simulink model "Sim_v18"  (Simulink 8.5)
settings: Solver=ode4  StartTime=0.0  StopTime=300  FixedStep=Ts  RelTol=1e-3
PreLoadFcn:
  | Ts=0.1;
PostLoadFcn:
  | Ts=0.1;
InitFcn:
  | Ts=0.1;
StartFcn:
  | Ts=0.1;
values from neighbouring files (symbols this model uses):
  ctrl_idx = strToIdx(actStr,loadNames)    [Driver_13NFbalanced.m]    (also in Driver_13NFunbalanced.m; Driver_4NFunbalanced.m; Driver_AL0001.m; Driver_Adam.m)
  dbc_idx = strToIdx(dbcStr,loadNames)    [Driver_13NFbalanced.m]    (also in Driver_13NFunbalanced.m; Driver_4NFunbalanced.m; Driver_AL0001.m; Driver_Adam.m)
  Ki_vang = zeros(r,1)    [Driver_4NFunbalanced.m]    (also in ZNset.m = 0.5*Ku/Tu; ZNtune.m = 0; afunc.m; computeK_ZN.m = zeros(1,r))
  Ki_vmag = [f2*ones(3,1); f3*ones(3,1)]    [Driver_4NFunbalanced.m]    (also in ZNset.m = 0.5*Ku/Tu; ZNtune.m = 0; afunc.m = zeros(r,1); computeK_ZN.m = zeros(1,r))
  Kp_vang = zeros(r,1)    [Driver_4NFunbalanced.m]    (also in ZNset.m = 0.4*Ku; ZNtune.m = 0.17; afunc.m; computeK_ZN.m = zeros(1,r))
  Kp_vmag = zeros(r,1)    [Driver_4NFunbalanced.m]    (also in ZNset.m = 0.4*Ku; ZNtune.m = 9.5; afunc.m; computeK_ZN.m = zeros(1,r))
  meas_idx = strToIdx(measStr,busNames)    [Driver_13NFbalanced.m]    (also in Driver_13NFunbalanced.m; Driver_4NFunbalanced.m; Driver_AL0001.m; Driver_Adam.m)
  Sbase = 500    [computePU.m]
  Sinv = 600    [Constraints_update.m]    (also in Driver_13NFbalanced.m = repmat(Sinv_str,1,length(ctrl_idx)/2); Driver_13NFunbalanced.m = repmat(Sinv_str,1,length(ctrl_idx)/2); Driver_4NFunbalanced.m = repmat(Sinv_str,1,length(ctrl_idx)/2); Driver_AL0001.m = repmat(Sinv_str,1,length(ctrl_idx)/2))
  V1base = V1_ph    [computePU.m]
  vang_init_actual = vang_new(4,:)    [Driver_13NFbalanced.m]    (also in Driver_13NFunbalanced.m = vang_new(40,:); Driver_4NFunbalanced.m = vang_new(40,:); Driver_AL0001.m = vang_new(40,:); Driver_Adam.m)
  Vmag_ctrlStart = 60    [Driver_4NFunbalanced.m]    (also in afunc.m = 5; computeK_ZN.m = 5; computeK_ZNplus.m = 5; computeK_way3.m = 5)
  vmag_init_actual = vmag_new(4,:)    [Driver_13NFbalanced.m]    (also in Driver_13NFunbalanced.m = vmag_new(40,:); Driver_4NFunbalanced.m = vmag_new(40,:); Driver_AL0001.m = vmag_new(40,:); Driver_Adam.m)
libraries: opal_lib x2, rtlab x2, rtlab_phasor x1
settings Model: Creator=Jaimie.Swartz  LastModifiedBy=Jaimie.Swartz
settings SolverCC: AlgebraicLoopSolver=LineSearch
settings DataIOCC: SignalLogging=off  DSMLogging=off  VisualizeSimOutput=off
settings DebuggingCC: SolverPrmCheckMsg=warning  FcnCallInpInsideContextMsg=EnableAllAsWarning
settings ConfigurationSet: Description=SimMechanics 2G

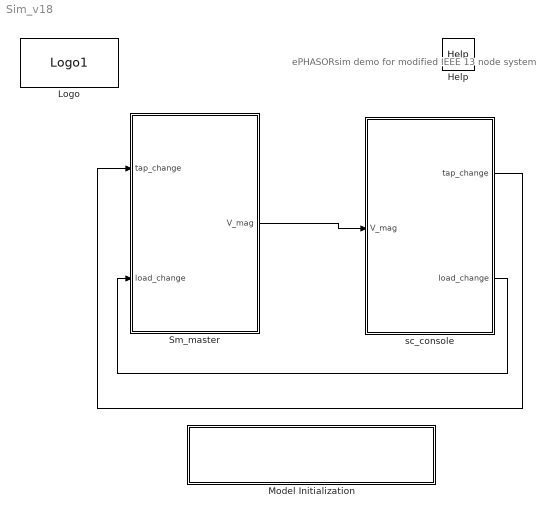
== system Sim_v18 ==
  note: ePHASORsim demo for
      | modified IEEE 13 node system
  Help : opal_lib/Help  docfile=../help/ePH_IEEE13.html
  Logo : opal_lib/Logo1  vide=[]
  Model Initialization : Subsystem  mask(Model Functions){InitFcnX=Ts=0.1;, prel=on, posl=on, inif=on, strf=on}
      mask prompts: InitFcnX "Initialisation"; prel "Preload Function"; posl "PostLoad Function"; inif "InitFcn"; strf "StartFcn"
      mask init:
      | currentBlock = gcb;
      | root = bdroot(currentBlock);
      | 
      | if ~strcmp(get_param(root,'BlockDiagramType'),'library')
      |     if prel==1
      |         set_param(root, 'PreLoadFcn', InitFcnX);
      |     else
      |         set_param(root, 'PreLoadFcn', '');
      |     end
      |     if inif==1
      |         set_param(root, 'InitFcn', InitFcnX);
      |     else
      |         set_param(root, 'InitFcn', '');
      |     end
      |     if strf==1
      |         set_param(root, 'StartFcn', InitFcnX);
      |     else
      |         set_param(root, 'StartFcn', '');
      |     end
      |     if posl==1
      |         set_param(root, 'PostLoadFcn', InitFcnX);
      |     else
      |         set_param(root, 'PostLoadFcn', '');
      |     end
      | end
      | 
      | pos = get_param(currentBlock, 'Position');
      | width = pos(3) - pos(1); height = pos(4) - pos(2);
      | txt = [ upper(root) '\n' '- InitFcn. . . . . '  get_param(root, 'InitFcn') ];
      settings: CopyFcn=set_param(gcb,'LinkStatus','none')
      mask Display: text(5, height*0.5, txt, 'horizontalAlignment', 'left', 'verticalAlignment', 'middle') ;
  Sm_master : Subsystem
  sc_console : Subsystem
  wires:
  Sm_master/1(V_mag) -> sc_console/1(V_mag)
  sc_console/1(tap_change) -> Sm_master/1(tap_change)
  sc_console/2(load_change) -> Sm_master/2(load_change)

== system Sim_v18/Model Initialization ==

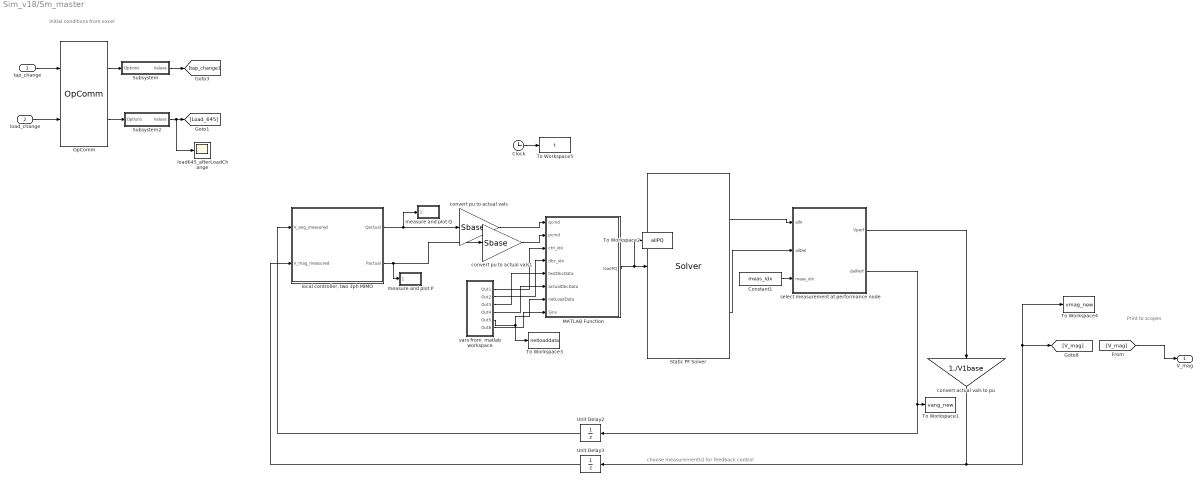
== system Sim_v18/Sm_master ==
  note: Initial conditions from excel
  note: choose measurement(s) for feedback control
  note: Print to scopes
  tap_change : Inport
  load_change : Inport  Port=2
  Clock : Clock
  Constant1 : Constant  Value=meas_idx
  MATLAB Function : MATLAB Function  TreatAsAtomicUnit=on
  OpComm : rtlab/OpComm  nbport=2  groupe_acq=1  subsys_rate=0  st=0  Synchronization=on  Interpolation=on  Threshold=1.0  Missed_Data=off  Sim_Time=off  Samples=off  dynSigOut=off  from_console=1  warning_done=off  writeOpCommFile=off  Offset=off
  Static PF Solver : rtlab_phasor/Solver  epname=System  extension=Excel  xls='impedMod_IEEE13.xls'  raw='4992b.raw'  dyr='4992b.dyr'  cyme='ieee13.sxst'  powerfactory='network.dgs'  builtin=on  cyme_pf=''  cyme_unbalanced=on  lazy_netlist=on  capidir='CAPI'  fmudir='FMU'  capiprefix=capicomp_  fmuprefix=fmucomp_  logging=off  sim_mode=Power-flow and dynamic simulation  pf_max_it=100  pf_tol_v=0.00000001  pf_flat_start=off  pf_smart_start=off  pf_export=on  np=1  exporty=off  dt=Ts  optim_threads=off  perflog_on=off  script_activate_postinit=off  script_postinit_name=''
  Subsystem : Subsystem
  Subsystem2 : Subsystem
  To Workspace1 : ToWorkspace  VariableName=vang_new  SampleTime=-1
      settings: Save2DSignal=2-D array (concatenate along first dimension)
  To Workspace2 : ToWorkspace  VariableName=allPQ  SampleTime=-1
      settings: Save2DSignal=2-D array (concatenate along first dimension)
  To Workspace3 : ToWorkspace  VariableName=netloaddata  SampleTime=-1
      settings: Save2DSignal=2-D array (concatenate along first dimension)
  To Workspace4 : ToWorkspace  VariableName=vmag_new  SampleTime=-1
      settings: Save2DSignal=2-D array (concatenate along first dimension)
  To Workspace5 : ToWorkspace  VariableName=t  SampleTime=-1
      settings: Save2DSignal=2-D array (concatenate along first dimension)
  Unit Delay2 : UnitDelay  InitialCondition=vang_init_actual  SampleTime=Ts
  Unit Delay3 : UnitDelay  InitialCondition=vmag_init_actual  SampleTime=Ts
  convert actual vals to pu : Gain  Gain=1./V1base
  convert pu to actual vals : Gain  Gain=Sbase
  convert pu to actual vals1 : Gain  Gain=Sbase
  load645_afterLoadChange : Scope
      settings: ShowLegends=on  YMin=0.94469  YMax=1.0518  SaveName=ScopeData17
  "local controller, two 3ph MIMO" : Subsystem
  measure and plot P : Subsystem
  measure and plot Q : Subsystem
  select measurement at performance node : MATLAB Function  TreatAsAtomicUnit=on
  vars from  matlab workspace : Subsystem
  V_mag : Outport
  wires:
  tap_change/1 -> OpComm/1
  load_change/1 -> OpComm/2
  [V_mag] -> V_mag/1
  OpComm/1 -> Subsystem/1(Options)
  OpComm/2 -> Subsystem2/1(Options)
  Subsystem/1(Values) -> [tap_change]
  Subsystem2/1(Values) -> load645_afterLoadChange/1, [Load_645]
  convert actual vals to pu/1 -> Unit Delay3/1, To Workspace4/1, [V_mag]
  Unit Delay2/1 -> "local controller, two 3ph MIMO"/1(V_ang_measured)
  Unit Delay3/1 -> "local controller, two 3ph MIMO"/2(V_mag_measured)
  Static PF Solver/1 -> select measurement at performance node/1(allV)
  Static PF Solver/2 -> select measurement at performance node/2(allDel)
  "local controller, two 3ph MIMO"/1(Qactual) -> convert pu to actual vals/1, measure and plot Q/1(Qactual)
  "local controller, two 3ph MIMO"/2(Pactual) -> measure and plot P/1(Pactual), convert pu to actual vals1/1
  MATLAB Function/1(loadPQ) -> To Workspace2/1, Static PF Solver/1
  select measurement at performance node/1(Vperf) -> convert actual vals to pu/1
  select measurement at performance node/2(delPerf) -> Unit Delay2/1, To Workspace1/1
  vars from  matlab workspace/1(Out1) -> MATLAB Function/3(ctrl_idx)
  vars from  matlab workspace/2(Out2) -> MATLAB Function/4(dbc_idx)
  Constant1/1 -> select measurement at performance node/3(meas_idx)
  vars from  matlab workspace/5(Out5) -> To Workspace3/1, MATLAB Function/7(netLoadData)
  convert pu to actual vals/1 -> MATLAB Function/1(qcmd)
  convert pu to actual vals1/1 -> MATLAB Function/2(pcmd)
  Clock/1 -> To Workspace5/1
  vars from  matlab workspace/3(Out3) -> MATLAB Function/5(testDbcData)
  vars from  matlab workspace/4(Out4) -> MATLAB Function/6(actualDbcData)
  vars from  matlab workspace/6(Out6) -> MATLAB Function/8(Sinv)

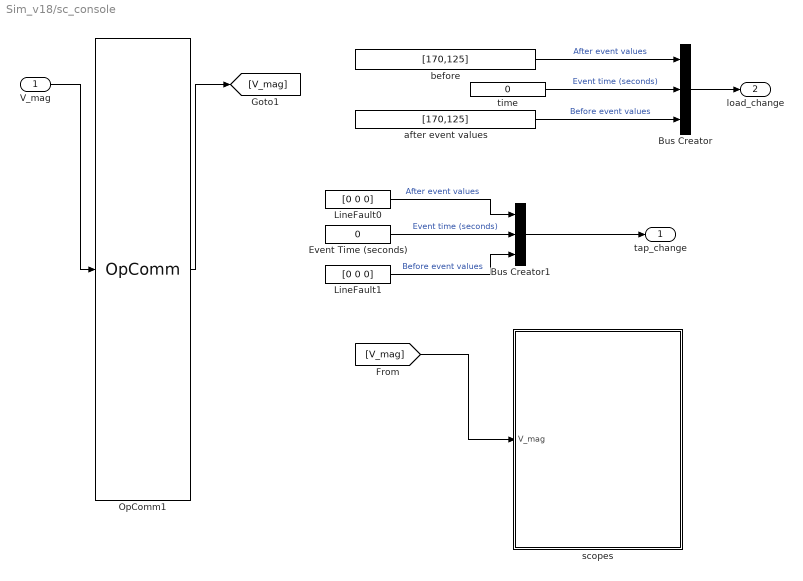
== system Sim_v18/sc_console ==
  V_mag : Inport
  Bus Creator : BusCreator  Inputs=3
  Bus Creator1 : BusCreator  Inputs=3
  Event Time (seconds) : Constant  Value=0
  LineFault0 : Constant  Value=[0 0 0]
  LineFault1 : Constant  Value=[0 0 0]
  OpComm1 : rtlab/OpComm  nbport=1  groupe_acq=1  subsys_rate=0  st=0  Synchronization=on  Interpolation=on  Threshold=1.0  Missed_Data=off  Sim_Time=off  Samples=off  dynSigOut=off  from_console=0  warning_done=off  writeOpCommFile=off  Offset=off
  after event values : Constant  Value=[170,125]
  before : Constant  Value=[170,125]
  scopes : Subsystem
  time : Constant  Value=0
  tap_change : Outport
  load_change : Outport  Port=2
  wires:
  V_mag/1 -> OpComm1/1
  OpComm1/1 -> [V_mag]
  time/1 -> Bus Creator/2  "Event time (seconds)"
  Bus Creator/1 -> load_change/1
  LineFault0/1 -> Bus Creator1/1  "After event values"
  LineFault1/1 -> Bus Creator1/3  "Before event values"
  Event Time (seconds)/1 -> Bus Creator1/2  "Event time (seconds)"
  Bus Creator1/1 -> tap_change/1
  before/1 -> Bus Creator/1  "After event values"
  after event values/1 -> Bus Creator/3  "Before event values"
  [V_mag] -> scopes/1(V_mag)

== system Sim_v18/Sm_master/Subsystem ==
  Options : Inport
  Bus Selector : BusSelector  OutputSignals=After event values,Event time (seconds),Before event values
  Clock : Clock
  Constant : Constant  Value=Ts/2
  Relational Operator : RelationalOperator  OutDataTypeStr=boolean
  Scope : Scope
  Sum : Sum  Inputs=|+-
  Switch : Switch  Threshold=0.5
  Values : Outport
  wires:
  Clock/1 -> Scope/1, Relational Operator/1
  Constant/1 -> Sum/2
  Sum/1 -> Relational Operator/2
  Bus Selector/2 -> Sum/1  "<Event time (seconds)>"
  Relational Operator/1 -> Switch/2
  Bus Selector/3 -> Switch/3  "<Before event values>"
  Bus Selector/1 -> Switch/1  "<After event values>"
  Switch/1 -> Values/1
  Options/1 -> Bus Selector/1

== system Sim_v18/Sm_master/Subsystem2 ==
  Options : Inport
  Bus Selector : BusSelector  OutputSignals=After event values,Event time (seconds),Before event values
  Clock : Clock
  Constant : Constant  Value=Ts/2
  Relational Operator : RelationalOperator  OutDataTypeStr=boolean
  Scope1 : Scope
      settings: SaveName=ScopeData14
  Scope2 : Scope
      settings: SaveName=ScopeData15
  Scope5 : Scope
      settings: SaveName=ScopeData13
  Sum : Sum  Inputs=|+-
  Switch : Switch  Threshold=0.5
  Values : Outport
  wires:
  Clock/1 -> Relational Operator/1
  Constant/1 -> Sum/2
  Sum/1 -> Relational Operator/2
  Bus Selector/2 -> Sum/1  "<Event time (seconds)>"
  Relational Operator/1 -> Switch/2
  Bus Selector/3 -> Switch/3, Scope1/1  "<Before event values>"
  Bus Selector/1 -> Switch/1, Scope5/1  "<After event values>"
  Switch/1 -> Values/1, Scope2/1
  Options/1 -> Bus Selector/1

== system Sim_v18/Sm_master/local controller, two 3ph MIMO ==
  note: P>Vang
  note: Q>Vang
  note: Q>Vmag
  note: P>Vmag
  V_ang_measured : Inport
  V_mag_measured : Inport  Port=2
  Sum2 : Sum  Inputs=+-
  Sum3 : Sum  Inputs=+-
  U >> Vang control : Subsystem
  U >> Vmag control : Subsystem
  satInd : Scope  NumInputPorts=2
      settings: ShowLegends=on  YMin=-1.4375~-5  YMax=0.9375~5  SaveName=ScopeData4
  sw1 : ManualSwitch
  sw2 : ManualSwitch  CurrentSetting=0
  Qactual : Outport
  Pactual : Outport  Port=2
  wires:
  sw1/1 -> Sum2/2, Qactual/1, Sum2/1
  U >> Vmag control/1(Unew) -> sw2/1, sw1/1  "Vmag"
  U >> Vang control/1(Unew) -> sw2/2, sw1/2  "Vang"
  V_mag_measured/1 -> U >> Vmag control/1(V_mag_measured)
  V_ang_measured/1 -> U >> Vang control/1(V_ang_measured)
  Sum2/1 -> satInd/1, U >> Vmag control/2(satIndicator)  "zero if unsaturated, pos if saturated"
  Sum3/1 -> U >> Vang control/2(satIndicator), satInd/2
  sw2/1 -> Sum3/2, Pactual/1, Sum3/1

== system Sim_v18/Sm_master/measure and plot P ==
  Pactual : Inport
  negate for aesthetic  sign convention2 : Gain  Gain=-1
  print2 : ToWorkspace  VariableName=pnew  SampleTime=-1
      settings: Save2DSignal=2-D array (concatenate along first dimension)
  wires:
  Pactual/1 -> negate for aesthetic  sign convention2/1
  negate for aesthetic  sign convention2/1 -> print2/1

== system Sim_v18/Sm_master/measure and plot Q ==
  Qactual : Inport
  negate for aesthetic  sign convention2 : Gain  Gain=-1
  print1 : ToWorkspace  VariableName=qnew  SampleTime=-1
      settings: Save2DSignal=2-D array (concatenate along first dimension)
  wires:
  Qactual/1 -> negate for aesthetic  sign convention2/1
  negate for aesthetic  sign convention2/1 -> print1/1

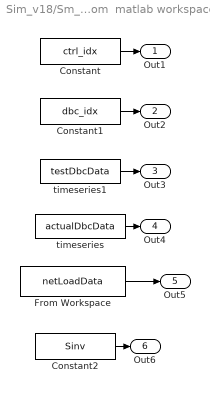
== system Sim_v18/Sm_master/vars from  matlab workspace ==
  Constant : Constant  Value=ctrl_idx
  Constant1 : Constant  Value=dbc_idx
  Constant2 : Constant  Value=Sinv
  From Workspace : FromWorkspace  VariableName=netLoadData  SampleTime=0
  timeseries : FromWorkspace  VariableName=actualDbcData  SampleTime=0
  timeseries1 : FromWorkspace  VariableName=testDbcData  SampleTime=0
  Out1 : Outport
  Out2 : Outport  Port=2
  Out3 : Outport  Port=3
  Out4 : Outport  Port=4
  Out5 : Outport  Port=5
  Out6 : Outport  Port=6
  wires:
  Constant/1 -> Out1/1
  Constant1/1 -> Out2/1
  From Workspace/1 -> Out5/1
  timeseries1/1 -> Out3/1
  timeseries/1 -> Out4/1
  Constant2/1 -> Out6/1

== system Sim_v18/sc_console/scopes ==
  note: for now just output everything to one scope
  V_mag : Inport
  Mag_bus_675 : Scope
      settings: YMin=0.92  YMax=1.07  SaveName=ScopeData6
  wires:
  V_mag/1 -> Mag_bus_675/1

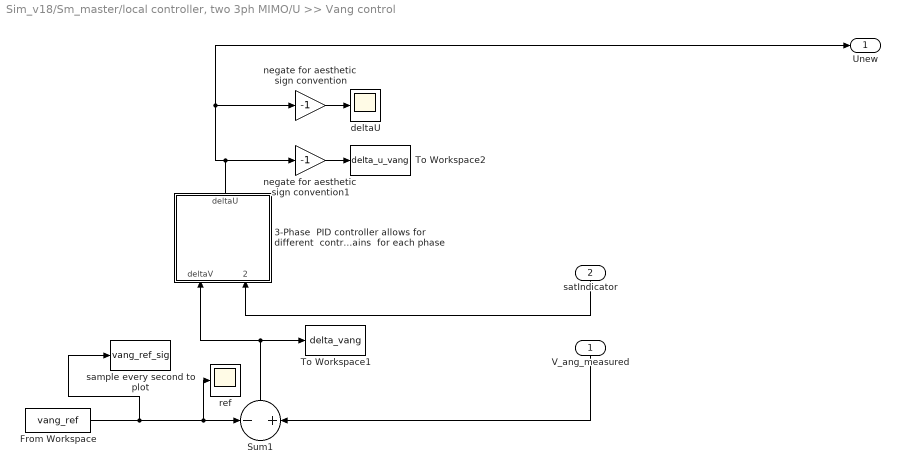
== system Sim_v18/Sm_master/local controller, two 3ph MIMO/U >> Vang control ==
  V_ang_measured : Inport
  satIndicator : Inport  Port=2
  3-Phase  PID controller allows for different  controller gains  for each phase : Subsystem
  From Workspace : FromWorkspace  VariableName=vang_ref  OutDataTypeStr=double  SampleTime=0
  Sum1 : Sum  Inputs=-|+
  To Workspace1 : ToWorkspace  VariableName=delta_vang  SampleTime=-1
  To Workspace2 : ToWorkspace  VariableName=delta_u_vang  SampleTime=-1
  deltaU : Scope
      settings: ShowLegends=on  YMin=-1.4375  YMax=0.9375
  negate for aesthetic  sign convention : Gain  Gain=-1
  negate for aesthetic  sign convention1 : Gain  Gain=-1
  ref : Scope
      settings: ShowLegends=on  YMin=-1.4375  YMax=0.9375  SaveName=ScopeData24
  sample every second to plot : ToWorkspace  VariableName=vang_ref_sig  SampleTime=-1
  Unew : Outport
  wires:
  negate for aesthetic  sign convention/1 -> deltaU/1
  Sum1/1 -> 3-Phase  PID controller allows for different  controller gains  for each phase/1(deltaV), To Workspace1/1
  3-Phase  PID controller allows for different  controller gains  for each phase/1(deltaU) -> Unew/1, negate for aesthetic  sign convention/1, negate for aesthetic  sign convention1/1
  negate for aesthetic  sign convention1/1 -> To Workspace2/1
  V_ang_measured/1 -> Sum1/2
  From Workspace/1 -> sample every second to plot/1, ref/1, Sum1/1
  satIndicator/1 -> 3-Phase  PID controller allows for different  controller gains  for each phase/2(satIndicator)

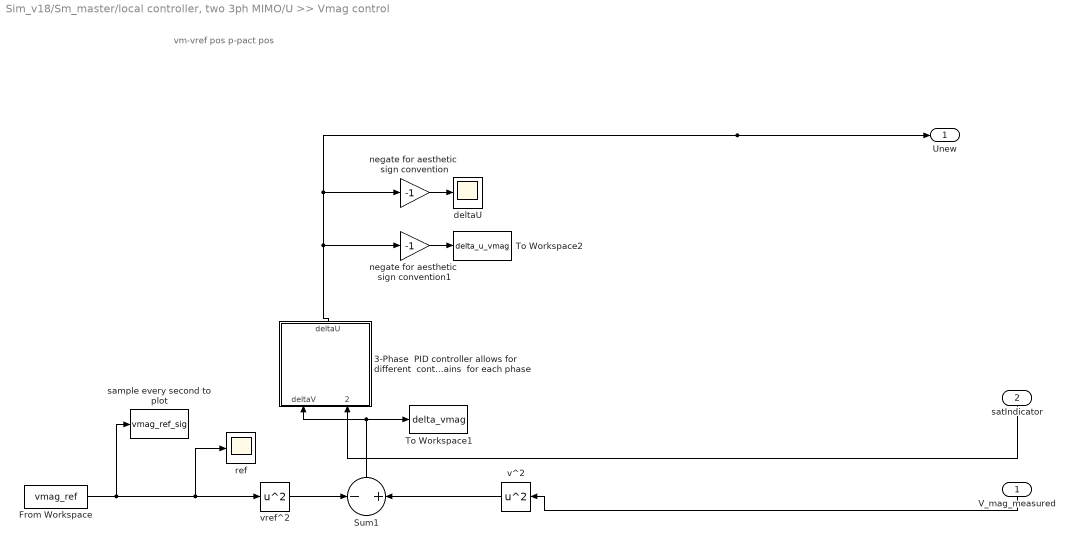
== system Sim_v18/Sm_master/local controller, two 3ph MIMO/U >> Vmag control ==
  note: vm-vref pos
      | p-pact pos
  V_mag_measured : Inport
  satIndicator : Inport  Port=2
  3-Phase  PID controller allows for different  controller gains  for each phase : Subsystem
  From Workspace : FromWorkspace  VariableName=vmag_ref  SampleTime=0
  Sum1 : Sum  Inputs=-|+
  To Workspace1 : ToWorkspace  VariableName=delta_vmag  SampleTime=-1
  To Workspace2 : ToWorkspace  VariableName=delta_u_vmag  SampleTime=-1
  deltaU : Scope
      settings: ShowLegends=on  YMin=-1.4375  YMax=0.9375
  negate for aesthetic  sign convention : Gain  Gain=-1
  negate for aesthetic  sign convention1 : Gain  Gain=-1
  ref : Scope
      settings: ShowLegends=on  YMin=-1.4375  YMax=0.9375  SaveName=ScopeData23
  sample every second to plot : ToWorkspace  VariableName=vmag_ref_sig  SampleTime=-1
  v^2 : Math  Operator=square  OutputSignalType=real  SaturateOnIntegerOverflow=on
  vref^2 : Math  Operator=square  OutputSignalType=real  SaturateOnIntegerOverflow=on
  Unew : Outport
  wires:
  V_mag_measured/1 -> v^2/1
  vref^2/1 -> Sum1/1
  negate for aesthetic  sign convention/1 -> deltaU/1
  v^2/1 -> Sum1/2
  Sum1/1 -> 3-Phase  PID controller allows for different  controller gains  for each phase/1(deltaV), To Workspace1/1
  3-Phase  PID controller allows for different  controller gains  for each phase/1(deltaU) -> negate for aesthetic  sign convention1/1, Unew/1, negate for aesthetic  sign convention/1
  negate for aesthetic  sign convention1/1 -> To Workspace2/1
  From Workspace/1 -> sample every second to plot/1, ref/1, vref^2/1
  satIndicator/1 -> 3-Phase  PID controller allows for different  controller gains  for each phase/2(satIndicator)

== system Sim_v18/Sm_master/local controller, two 3ph MIMO/U >> Vang control/3-Phase  PID controller allows for different  controller gains  for each phase ==
  deltaV : Inport
  satIndicator : Inport  Port=2
  Demux1 : Demux  Outputs=3
  Demux2 : Demux  Outputs=3
  Mux1 : Mux  Inputs=3
  "SISO PID controller, PhA1" : Subsystem
  "SISO PID controller, PhB1" : Subsystem
  "SISO PID controller, PhC1" : Subsystem
  To Workspace : ToWorkspace  VariableName=deltaU_mm  SaveFormat=Timeseries  SampleTime=-1
  deltaU : Outport
  wires:
  "SISO PID controller, PhB1"/1(U_phB) -> Mux1/2
  Mux1/1 -> To Workspace/1, deltaU/1
  "SISO PID controller, PhC1"/1(U_phC) -> Mux1/3
  Demux1/3 -> "SISO PID controller, PhC1"/1(deltaY_phC)
  Demux1/2 -> "SISO PID controller, PhB1"/1(deltaY_phB3)
  Demux1/1 -> "SISO PID controller, PhA1"/1(deltaY_phA3)
  deltaV/1 -> Demux1/1
  "SISO PID controller, PhA1"/1(U_phA) -> Mux1/1
  Demux2/1 -> "SISO PID controller, PhA1"/2(satIndicator)
  Demux2/2 -> "SISO PID controller, PhB1"/2(satIndicator)
  satIndicator/1 -> Demux2/1
  Demux2/3 -> "SISO PID controller, PhC1"/2(satIndicator)

== system Sim_v18/Sm_master/local controller, two 3ph MIMO/U >> Vmag control/3-Phase  PID controller allows for different  controller gains  for each phase ==
  deltaV : Inport
  satIndicator : Inport  Port=2
  Demux : Demux  Outputs=3
  Demux1 : Demux  Outputs=3
  Mux : Mux  Inputs=3
  "SISO PID controller, PhA" : Subsystem
  "SISO PID controller, PhB" : Subsystem
  "SISO PID controller, PhC" : Subsystem
  deltaU : Outport
  wires:
  "SISO PID controller, PhB"/1(U_phB) -> Mux/2
  Mux/1 -> deltaU/1
  "SISO PID controller, PhC"/1(U_phC) -> Mux/3
  Demux/3 -> "SISO PID controller, PhC"/1(deltaY_phC)
  Demux/2 -> "SISO PID controller, PhB"/1(deltaY_phB3)
  Demux/1 -> "SISO PID controller, PhA"/1(deltaY_phA)
  deltaV/1 -> Demux/1
  "SISO PID controller, PhA"/1(U_phA) -> Mux/1
  Demux1/1 -> "SISO PID controller, PhA"/2(satIndicator)
  Demux1/2 -> "SISO PID controller, PhB"/2(satIndicator)
  satIndicator/1 -> Demux1/1
  Demux1/3 -> "SISO PID controller, PhC"/2(satIndicator)

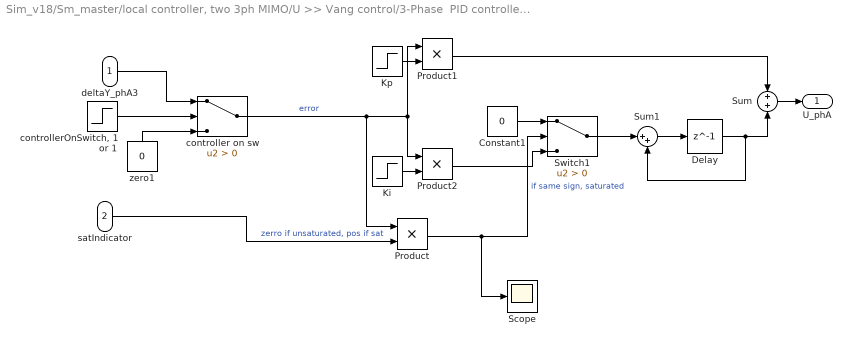
== system Sim_v18/Sm_master/local controller, two 3ph MIMO/U >> Vang control/3-Phase  PID controller allows for different  controller gains  for each phase/SISO PID controller, PhA1 ==
  deltaY_phA3 : Inport
  satIndicator : Inport  Port=2
  Constant1 : Constant  Value=0
  Delay : Delay  DelayLength=1  InitialCondition=0
  Ki : Step  Time=57  Before=Ki_vang(1)  After=Ki_vang(1)  SampleTime=Ts
  Kp : Step  Time=57  Before=Kp_vang(1)  After=Kp_vang(1)  SampleTime=Ts
  Product : Product
  Product1 : Product
  Product2 : Product
  Scope : Scope
      settings: SaveName=ScopeData5
  Sum : Sum
  Sum1 : Sum  Inputs=|++
  Switch1 : Switch  Criteria=u2 > Threshold
  controller on sw : Switch  Criteria=u2 > Threshold
  "controllerOnSwitch, 1 or 1" : Step  Time=Vmag_ctrlStart  SampleTime=0
  zero1 : Constant  Value=0
  U_phA : Outport
  wires:
  Constant1/1 -> Switch1/1
  Product2/1 -> Switch1/3
  Sum1/1 -> Delay/1
  Delay/1 -> Sum1/2, Sum/2
  Product1/1 -> Sum/1
  Switch1/1 -> Sum1/1
  Product/1 -> Scope/1, Switch1/2  "if same sign, saturated"
  Ki/1 -> Product2/2
  Kp/1 -> Product1/2
  controller on sw/1 -> Product1/1, Product2/1, Product/1  "error"
  "controllerOnSwitch, 1 or 1"/1 -> controller on sw/2
  deltaY_phA3/1 -> controller on sw/1
  zero1/1 -> controller on sw/3
  Sum/1 -> U_phA/1
  satIndicator/1 -> Product/2  "zerro if unsaturated, pos if sat"

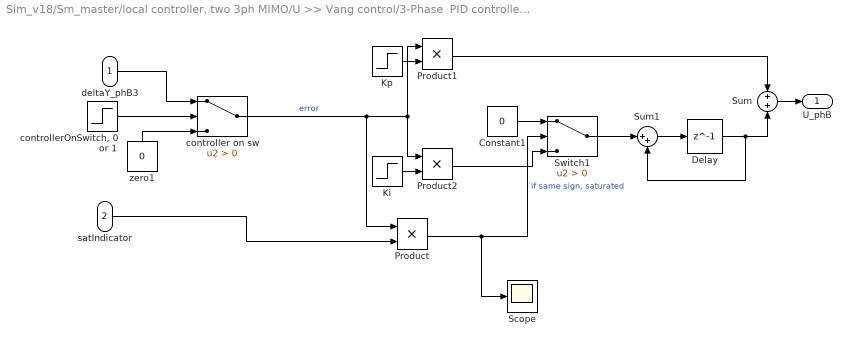
== system Sim_v18/Sm_master/local controller, two 3ph MIMO/U >> Vang control/3-Phase  PID controller allows for different  controller gains  for each phase/SISO PID controller, PhB1 ==
  deltaY_phB3 : Inport
  satIndicator : Inport  Port=2
  Constant1 : Constant  Value=0
  Delay : Delay  DelayLength=1  InitialCondition=0
  Ki : Step  Time=57  Before=Ki_vang(2)  After=Ki_vang(2)  SampleTime=Ts
  Kp : Step  Time=57  Before=Kp_vang(2)  After=Kp_vang(2)  SampleTime=Ts
  Product : Product
  Product1 : Product
  Product2 : Product
  Scope : Scope
      settings: YMin=-0.1  YMax=0.1  SaveName=ScopeData3
  Sum : Sum
  Sum1 : Sum  Inputs=|++
  Switch1 : Switch  Criteria=u2 > Threshold
  controller on sw : Switch  Criteria=u2 > Threshold
  "controllerOnSwitch, 0 or 1" : Step  Time=Vmag_ctrlStart  SampleTime=0
  zero1 : Constant  Value=0
  U_phB : Outport
  wires:
  Constant1/1 -> Switch1/1
  Product2/1 -> Switch1/3
  Sum1/1 -> Delay/1
  Delay/1 -> Sum1/2, Sum/2
  Product1/1 -> Sum/1
  Switch1/1 -> Sum1/1
  Product/1 -> Scope/1, Switch1/2  "if same sign, saturated"
  Ki/1 -> Product2/2
  Kp/1 -> Product1/2
  controller on sw/1 -> Product1/1, Product2/1, Product/1  "error"
  "controllerOnSwitch, 0 or 1"/1 -> controller on sw/2
  deltaY_phB3/1 -> controller on sw/1
  zero1/1 -> controller on sw/3
  Sum/1 -> U_phB/1
  satIndicator/1 -> Product/2

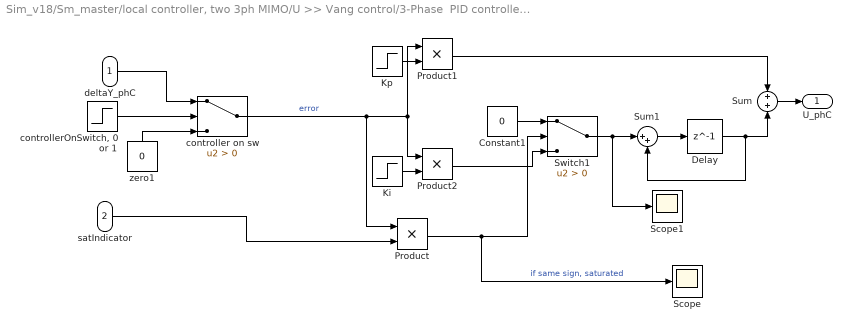
== system Sim_v18/Sm_master/local controller, two 3ph MIMO/U >> Vang control/3-Phase  PID controller allows for different  controller gains  for each phase/SISO PID controller, PhC1 ==
  deltaY_phC : Inport
  satIndicator : Inport  Port=2
  Constant1 : Constant  Value=0
  Delay : Delay  DelayLength=1  InitialCondition=0
  Ki : Step  Time=57  Before=Ki_vang(3)  After=Ki_vang(3)  SampleTime=Ts
  Kp : Step  Time=57  Before=Kp_vang(3)  After=Kp_vang(3)  SampleTime=Ts
  Product : Product
  Product1 : Product
  Product2 : Product
  Scope : Scope
      settings: SaveName=ScopeData10
  Scope1 : Scope
      settings: YMin=-0.1  YMax=0.1  SaveName=ScopeData22
  Sum : Sum
  Sum1 : Sum  Inputs=|++
  Switch1 : Switch  Criteria=u2 > Threshold
  controller on sw : Switch  Criteria=u2 > Threshold
  "controllerOnSwitch, 0 or 1" : Step  Time=Vmag_ctrlStart  SampleTime=0
  zero1 : Constant  Value=0
  U_phC : Outport
  wires:
  Constant1/1 -> Switch1/1
  Product2/1 -> Switch1/3
  Sum1/1 -> Delay/1
  Delay/1 -> Sum1/2, Sum/2
  Product1/1 -> Sum/1
  Switch1/1 -> Scope1/1, Sum1/1
  Product/1 -> Scope/1, Switch1/2  "if same sign, saturated"
  Ki/1 -> Product2/2
  Kp/1 -> Product1/2
  controller on sw/1 -> Product1/1, Product2/1, Product/1  "error"
  "controllerOnSwitch, 0 or 1"/1 -> controller on sw/2
  deltaY_phC/1 -> controller on sw/1
  zero1/1 -> controller on sw/3
  Sum/1 -> U_phC/1
  satIndicator/1 -> Product/2

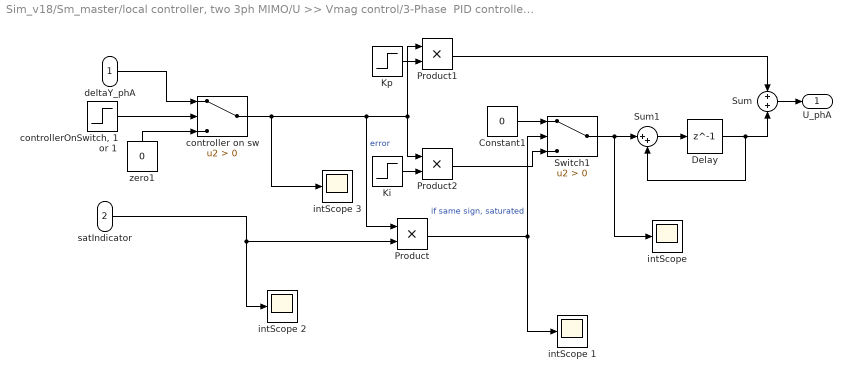
== system Sim_v18/Sm_master/local controller, two 3ph MIMO/U >> Vmag control/3-Phase  PID controller allows for different  controller gains  for each phase/SISO PID controller, PhA ==
  deltaY_phA : Inport
  satIndicator : Inport  Port=2
  Constant1 : Constant  Value=0
  Delay : Delay  DelayLength=1  InitialCondition=0
  Ki : Step  Time=57  Before=Ki_vmag(1)  After=Ki_vmag(1)  SampleTime=Ts
  Kp : Step  Time=57  Before=Kp_vmag(1)  After=Kp_vmag(1)  SampleTime=Ts
  Product : Product
  Product1 : Product
  Product2 : Product
  Sum : Sum
  Sum1 : Sum  Inputs=|++
  Switch1 : Switch  Criteria=u2 > Threshold
  controller on sw : Switch  Criteria=u2 > Threshold
  "controllerOnSwitch, 1 or 1" : Step  Time=Vmag_ctrlStart  SampleTime=0
  intScope {,1..3} (4 alike) : Scope
      "intScope " settings: YMin=-0.25  YMax=0.1  SaveName=ScopeData21
      intScope 1 settings: YMin=-0.1  YMax=0.1  SaveName=ScopeData25
      intScope 2 settings: YMin=-0.1  YMax=0.1  SaveName=ScopeData26
      intScope 3 settings: YMin=-0.1  YMax=0.1  SaveName=ScopeData27
  zero1 : Constant  Value=0
  U_phA : Outport
  wires:
  Constant1/1 -> Switch1/1
  Product2/1 -> Switch1/3
  Sum1/1 -> Delay/1
  Delay/1 -> Sum1/2, Sum/2
  Product1/1 -> Sum/1
  Switch1/1 -> "intScope "/1, Sum1/1
  Product/1 -> Switch1/2, intScope 1/1  "if same sign, saturated"
  Ki/1 -> Product2/2
  Kp/1 -> Product1/2
  controller on sw/1 -> intScope 3/1, Product1/1, Product2/1, Product/1  "error"
  "controllerOnSwitch, 1 or 1"/1 -> controller on sw/2
  deltaY_phA/1 -> controller on sw/1
  zero1/1 -> controller on sw/3
  Sum/1 -> U_phA/1
  satIndicator/1 -> intScope 2/1, Product/2

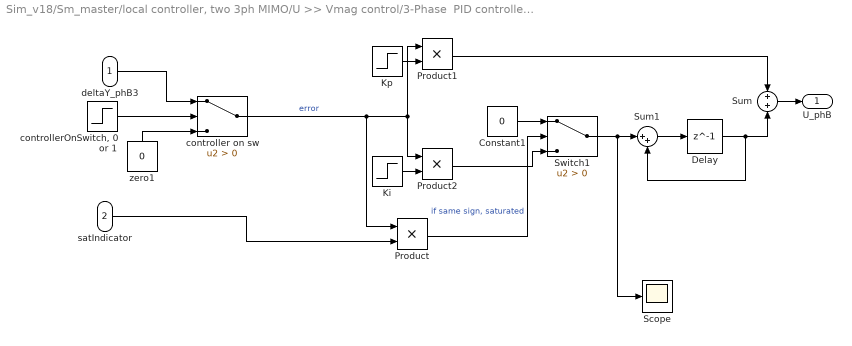
== system Sim_v18/Sm_master/local controller, two 3ph MIMO/U >> Vmag control/3-Phase  PID controller allows for different  controller gains  for each phase/SISO PID controller, PhB ==
  deltaY_phB3 : Inport
  satIndicator : Inport  Port=2
  Constant1 : Constant  Value=0
  Delay : Delay  DelayLength=1  InitialCondition=0
  Ki : Step  Time=57  Before=Ki_vmag(2)  After=Ki_vmag(2)  SampleTime=Ts
  Kp : Step  Time=57  Before=Kp_vmag(2)  After=Kp_vmag(2)  SampleTime=Ts
  Product : Product
  Product1 : Product
  Product2 : Product
  Scope : Scope
      settings: YMin=-0.1  YMax=0.1  SaveName=ScopeData3
  Sum : Sum
  Sum1 : Sum  Inputs=|++
  Switch1 : Switch  Criteria=u2 > Threshold
  controller on sw : Switch  Criteria=u2 > Threshold
  "controllerOnSwitch, 0 or 1" : Step  Time=Vmag_ctrlStart  SampleTime=0
  zero1 : Constant  Value=0
  U_phB : Outport
  wires:
  Constant1/1 -> Switch1/1
  Product2/1 -> Switch1/3
  Sum1/1 -> Delay/1
  Delay/1 -> Sum1/2, Sum/2
  Product1/1 -> Sum/1
  Switch1/1 -> Scope/1, Sum1/1
  Product/1 -> Switch1/2  "if same sign, saturated"
  Ki/1 -> Product2/2
  Kp/1 -> Product1/2
  controller on sw/1 -> Product1/1, Product2/1, Product/1  "error"
  "controllerOnSwitch, 0 or 1"/1 -> controller on sw/2
  deltaY_phB3/1 -> controller on sw/1
  zero1/1 -> controller on sw/3
  Sum/1 -> U_phB/1
  satIndicator/1 -> Product/2

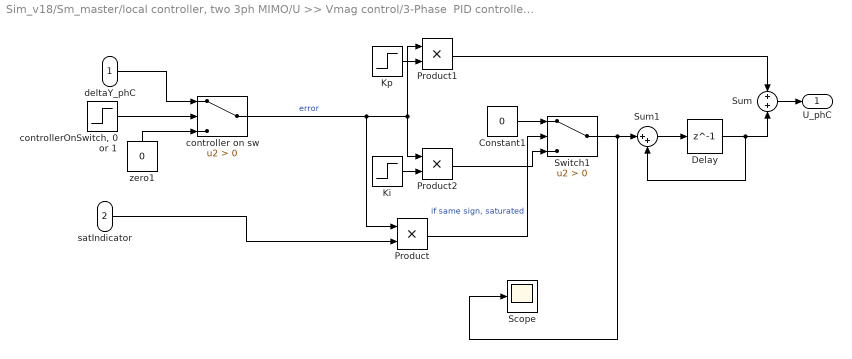
== system Sim_v18/Sm_master/local controller, two 3ph MIMO/U >> Vmag control/3-Phase  PID controller allows for different  controller gains  for each phase/SISO PID controller, PhC ==
  deltaY_phC : Inport
  satIndicator : Inport  Port=2
  Constant1 : Constant  Value=0
  Delay : Delay  DelayLength=1  InitialCondition=0
  Ki : Step  Time=57  Before=Ki_vmag(3)  After=Ki_vmag(3)  SampleTime=Ts
  Kp : Step  Time=57  Before=Kp_vmag(3)  After=Kp_vmag(3)  SampleTime=Ts
  Product : Product
  Product1 : Product
  Product2 : Product
  Scope : Scope
      settings: YMin=-0.1  YMax=0.1  SaveName=ScopeData10
  Sum : Sum
  Sum1 : Sum  Inputs=|++
  Switch1 : Switch  Criteria=u2 > Threshold
  controller on sw : Switch  Criteria=u2 > Threshold
  "controllerOnSwitch, 0 or 1" : Step  Time=Vmag_ctrlStart  SampleTime=0
  zero1 : Constant  Value=0
  U_phC : Outport
  wires:
  Constant1/1 -> Switch1/1
  Product2/1 -> Switch1/3
  Sum1/1 -> Delay/1
  Delay/1 -> Sum1/2, Sum/2
  Product1/1 -> Sum/1
  Switch1/1 -> Scope/1, Sum1/1
  Product/1 -> Switch1/2  "if same sign, saturated"
  Ki/1 -> Product2/2
  Kp/1 -> Product1/2
  controller on sw/1 -> Product1/1, Product2/1, Product/1  "error"
  "controllerOnSwitch, 0 or 1"/1 -> controller on sw/2
  deltaY_phC/1 -> controller on sw/1
  zero1/1 -> controller on sw/3
  Sum/1 -> U_phC/1
  satIndicator/1 -> Product/2

== matlab function Sm_master/select measurement at performance node ==
  data: Vperf output double; allV input double; allDel input double; delPerf output double; meas_idx input double
function [Vperf,delPerf]=selectMeas(allV,allDel,meas_idx)
% use measStr,nodeNames from workspace
    Vperf=allV(meas_idx);
    delPerf=allDel(meas_idx);
end

== matlab function Sm_master/MATLAB Function ==
  data: qcmd input double; pcmd input double; loadPQ output double; ctrl_idx input double; dbc_idx input double; testDbcData input double; actualDbcData input double; netLoadData input double; Sinv input double
function loadPQ =updatePows(qcmd,pcmd,ctrl_idx,dbc_idx,testDbcData,actualDbcData,netLoadData, Sinv)
% netLoadData, dbcData, and k are timeseries, fed once by one for each timestep
% ctrl_idx and dbc_idx are constant
    % inputs: 
        % k is current timestep
        % 3x1 vectors of unadjusted actuation, as if have 1 actuator and it's located at the perf node 
    % inputs: rx1 vectors of powers at all nodes 
        % r is number of phases across all nodes, i.e. the dim of the pin
        % vector input to RTlab solve
       
   %% actuation signal sent from controller to devices
   %% Devices actuate here:
    % Device enforces basic inv limit by moving operating piont to closest
    % point on the inv circle
    pact=zeros(3,3); qact=zeros(3,3); % initialize, TEMP, assume single actuator is on 3 phases
    for i=1:3 % across phases, TEMP, assuming the single actuator is on 3 phases
        if pcmd(i)^2+qcmd(i)^2>Sinv(i)^2
            pact(i)=pcmd(i)*Sinv(i)/(sqrt(pcmd(i)^2+qcmd(i)^2))
            qact(i)=pcmd(i)*Sinv(i)/(sqrt(pcmd(i)^2+qcmd(i)^2))
        else
            pact(i)=pcmd(i);
            qact(i)=qcmd(i);
        end
    end
%%
    PQact=[pact(1) qact(1) pact(2) qact(2) pact(3) qact(3)]';
    % TEMP^ not an elegant fix, assumes single actuator
    %loadPQ=zeros(size(netLoadData));
    loadPQ=netLoadData; % P&Q, ordered according to loadNames
    loadPQ(ctrl_idx)=loadPQ(ctrl_idx)+PQact+testDbcData; 
    loadPQ(dbc_idx)=loadPQ(dbc_idx)+actualDbcData;

end
